simulink model "three_phase_FullyControlled_rectifyer"  (R2022a)
settings: Solver=VariableStepAuto  StartTime=0.0  StopTime=0.04  RelTol=1e-3
libraries: spsThyristorLib x6, spsVoltageMeasurementLib x5, spsACVoltageSourceLib x3, spsSeriesRLCBranchLib x1, spsCurrentMeasurementLib x1, spsGroundLib x1, spspowerguiLib x1
settings Model: Creator=HP  LastModifiedBy=P.O.M.G
settings SolverCC: AlgebraicLoopSolver=TrustRegion
settings DataIOCC: ReturnWorkspaceOutputs=off
settings OptimizationCC: LifeSpan=inf
settings DebuggingCC: UnconnectedInputMsg=warning  UnconnectedOutputMsg=warning  UnconnectedLineMsg=warning  SFExecutionAtInitializationDiag=none  SFMachineParentedDataDiag=warning  ArithmeticOperatorsInVariantConditions=warning
settings SFSimCC: SimUseLocalCustomCode=off  CustomCodeUndefinedFunction=UseInterfaceOnly
settings RTWCC: RTWUseLocalCustomCode=off
settings CodeAppCC: StateflowObjectComments=on
settings SimscapeCC: SimscapeNormalizeSystem=off

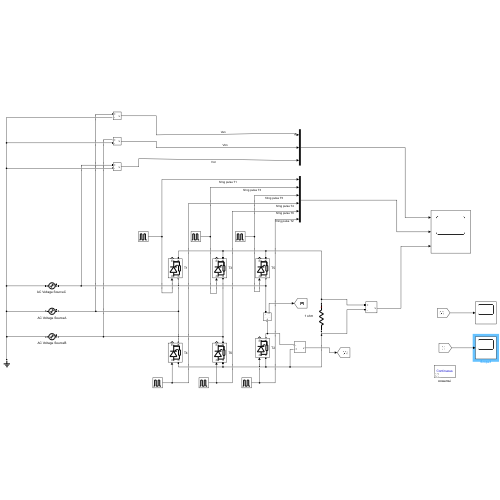
[thumbnail: Simulink's stored preview of the top-level diagram]
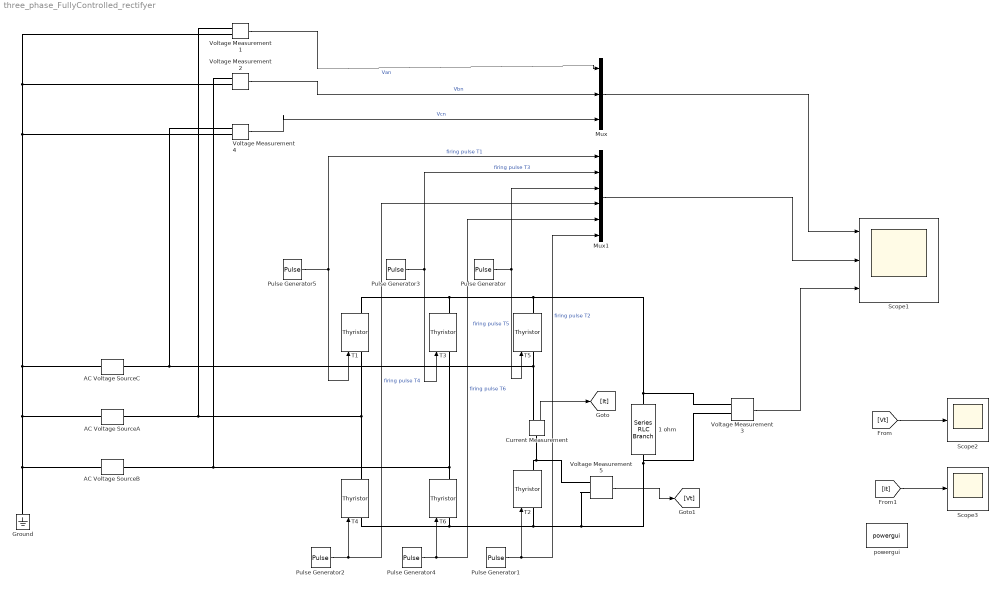
== system three_phase_FullyControlled_rectifyer ==
  "1 ohm " : spsSeriesRLCBranchLib/Series RLC Branch  LConnTagsString=__new0  RConnTagsString=__new0  BranchType=R  Resistance=100  Inductance=10  SetiL0=off  InitialCurrent=0  Capacitance=1e-6  Setx0=off  InitialVoltage=0  Measurements=None
  AC Voltage SourceA : spsACVoltageSourceLib/AC Voltage Source  Amplitude=308  Phase=0  Frequency=50  SampleTime=1e-5  Measurements=None  BusType=swing  Pref=10e3  Qref=0  Qmin=-inf  Qmax=+inf
  AC Voltage SourceB : spsACVoltageSourceLib/AC Voltage Source  Amplitude=308  Phase=240  Frequency=50  SampleTime=1e-5  Measurements=None  BusType=swing  Pref=10e3  Qref=0  Qmin=-inf  Qmax=+inf
  "AC Voltage SourceC " : spsACVoltageSourceLib/AC Voltage Source  Amplitude=308  Phase=120  Frequency=50  SampleTime=1e-5  Measurements=None  BusType=swing  Pref=10e3  Qref=0  Qmin=-inf  Qmax=+inf
  Current Measurement : spsCurrentMeasurementLib/Current Measurement  PhasorSimulation=off  OutputType=Complex  PSBequivalent=0
  Ground : spsGroundLib/Ground  LConnTagsString=a
  Mux : Mux  Inputs=3
  Mux1 : Mux  Inputs=6
  Pulse Generator : DiscretePulseGenerator  PulseType=Time based  Amplitude=2  Period=0.02  PulseWidth=5  PhaseDelay=0.014167
  Pulse Generator1 : DiscretePulseGenerator  PulseType=Time based  Amplitude=2  Period=0.02  PulseWidth=5  PhaseDelay=0.004167
  Pulse Generator2 : DiscretePulseGenerator  PulseType=Time based  Amplitude=2  Period=0.02  PulseWidth=5  PhaseDelay=0.010833
  Pulse Generator3 : DiscretePulseGenerator  PulseType=Time based  Amplitude=2  Period=0.02  PulseWidth=5  PhaseDelay=0.0075
  Pulse Generator4 : DiscretePulseGenerator  PulseType=Time based  Amplitude=2  Period=0.02  PulseWidth=5  PhaseDelay=0.0175
  Pulse Generator5 : DiscretePulseGenerator  PulseType=Time based  Amplitude=2  Period=0.02  PulseWidth=5  PhaseDelay=0.000833
  Scope1 : Scope  NumInputPorts=3
  Scope2 : Scope
  Scope3 : Scope
  T{1..6} (6 alike) : spsThyristorLib/Thyristor  Ron=0.001  Lon=0  Vf=0.8  IC=0  Rs=500  Cs=250e-9  Measurements=on
  Voltage Measurement{1..5} (5 alike) : spsVoltageMeasurementLib/Voltage Measurement  PhasorSimulation=off  OutputType=Complex  PSBequivalent=0
  powergui : spspowerguiLib/powergui  Priority=1  SimulationMode=Continuous  SampleTime=50e-6  frequency=60  Iterations=50  frequencyindice=50  Pbase=100e6  ErrMax=1e-4  UnitsV=kV  UnitsW=MW  buscounter=0  FunctionMessages=off  echomessages=off  EnableUseOfTLC=off  CurrentSourceSwitches=off  DisableSnubberDevices=off  DisableRonSwitches=off  DisableVfSwitches=off  DisplayEquations=off  AutomaticDiscreteSolvers=off  SolverType=Tustin/Backward Euler (TBE)  Interpol=off  ExternalGateDelay=off  methode=off  Ts=100  x0status=blocks  SPID=off  SwTol=0  HookPort=off  NonlinearTolerance=1e-4  nMaxIteration=100  ContinueOnMaxIteration=off  RestoreLinks=warning  ResistiveCurrentMeasurement=off  Frange=[0:2:500]  Ylog=off  Xlog=on  ShowGrid=off  save=off  variable=ZData  structure=0  ZoomFFT=off  StartTime=0.0  cycles=1  DisplayStyle=1  fundamental=60  FreqAxis=off  MaxFrequency=1000  frequencyindicesteady=1  RmsSteady=1  display=off
  wires:
  Pulse Generator/1 -> Mux1/3, T5/1  "firing pulse T5"
  Pulse Generator1/1 -> T2/1, Mux1/6  "firing pulse T2"
  Pulse Generator2/1 -> T4/1, Mux1/4  "firing pulse T4"
  Pulse Generator3/1 -> Mux1/2, T3/1  "firing pulse T3"
  Pulse Generator4/1 -> T6/1, Mux1/5  "firing pulse T6"
  Pulse Generator5/1 -> Mux1/1, T1/1  "firing pulse T1"
  Voltage Measurement1/1 -> Mux/1  "Van"
  Voltage Measurement2/1 -> Mux/2  "Vbn"
  Voltage Measurement4/1 -> Mux/3  "Vcn"
  Voltage Measurement3/1 -> Scope1/3
  Mux1/1 -> Scope1/2
  Mux/1 -> Scope1/1
  [Vt] -> Scope2/1
  [It] -> Scope3/1
  Current Measurement/1 -> [It]
  Voltage Measurement5/1 -> [Vt]
  connections:
  Ground/LConn1 -- Voltage Measurement4/LConn2 -- Voltage Measurement2/LConn2 -- Voltage Measurement1/LConn2 -- "AC Voltage SourceC "/LConn1 -- AC Voltage SourceA/LConn1 -- AC Voltage SourceB/LConn1
  "AC Voltage SourceC "/RConn1 -- Voltage Measurement4/LConn1 -- T5/LConn1 -- Current Measurement/RConn1
  AC Voltage SourceA/RConn1 -- Voltage Measurement1/LConn1 -- T1/LConn1 -- T4/RConn1
  "1 ohm "/RConn1 -- Voltage Measurement5/LConn1 -- T4/LConn1 -- T6/LConn1 -- T2/LConn1 -- Voltage Measurement3/LConn2
  T5/RConn1 -- T1/RConn1 -- T3/RConn1 -- Voltage Measurement3/LConn1 -- "1 ohm "/LConn1
  T3/LConn1 -- Voltage Measurement2/LConn1 -- AC Voltage SourceB/RConn1 -- T6/RConn1
  T2/RConn1 -- Current Measurement/LConn1 -- Voltage Measurement5/LConn2
